simulink model "Hector_Simulation"  (R2023b)
settings: Solver=daessc  StartTime=0.0  StopTime=Tf  FixedStep=0.001  MaxStep=1e-3  RelTol=1e-2
model workspace (MATLAB code in the model file):
  | %% World Plane
  | plane_x = 20;
  | plane_y = 2;
  | plane_z = 0.05;
  | 
  | %% motor
  | %A1
  | motor_com = [0, -0.02,0];
  | motor_com_mirror = [0, 0.02,0];
  | 
  | motor_I = [0.00048,0.00071,0.00048];
  | motor_mass = 0.605;
  | 
  | %% Body
  | % Inertial
  | body_com_x = 0.0;
  | body_com_y = 0.0;
  | body_com_z = -0.0;
  | body_mass = 5.75;
  | body_ixx = 44350*1e-6;
  | body_ixy = 0.0;
  | body_ixz = 0.0;
  | body_iyy = 53149*1e-6;
  | body_iyz = 0.0;
  | body_izz = 21390*1e-6;
  | 
  | %% Hip 1
  | % joint
  | hip1_offset_x =0.0;
  | hip1_offset_y = 0.047;
  | hip1_offset_z = 0.1265;
  | % hip1_max = 15;
  | % hip1_min = -15;
  | hip1_velocity_max = 21;
  | hip1_torque_max = 33.5;
  | % Inertial
  | hip1_com_x = 0.0268;
  | hip1_com_y = -0.00315;
  | hip1_com_z = -0.0272;
  | hip1_mass = 0.173;
  | hip1_ixx = 0.00022;
  | hip1_ixy = 0.0;
  | hip1_ixz = 0.0;
  | hip1_iyy = 0.00024;
  | hip1_iyz = 0.0;
  | hip1_izz = 0.00016;
  | 
  | %% Hip 2
  | % joint
  | hip2_offset_x =0.053;
  | hip2_offset_y = 0.0185;
  | hip2_offset_z = 0.071;
  | % hip2_max = 15;
  | % hip2_min = -15;
  | hip2_velocity_max = 21;
  | hip2_torque_max = 33.5;
  | % Inertial
  | hip2_com_x = -0.0308;
  | hip2_com_y = -0.00942;
  | hip2_com_z = 0.0;
  | hip2_mass = 0.0722;
  | hip2_ixx = 0.0000422;
  | hip2_ixy = 0.0;
  | hip2_ixz = 0.0;
  | hip2_iyy = 0.000120;
  | hip2_iyz = 0.0;
  | hip2_izz = 0.0000708;
  | 
  | %% Thigh
  | % joint
  | thigh_offset_x =-0.06;
  | thigh_offset_y = 0.004;
  | thigh_offset_z = 0.0;
  | % thigh_max = 130;
  | % thigh_min = -45;
  | thigh_velocity_max = 21;
  | thigh_torque_max = 33.5;
  | % Inertial
  | thigh_com_x = -0.00143;
  | thigh_com_y = -0.02106;
  | thigh_com_z = -0.06115;
  | thigh_mass = 0.397;
  | thigh_ixx = 0.00197;
  | thigh_ixy = 0.0;
  | thigh_ixz = 0.0;
  | thigh_iyy = 0.00218;
  | thigh_iyz = 0.0;
  | thigh_izz = 0.00033;
  | 
  | ankle_motor_offset_x = 0;
  | ankle_motor_offset_y = 0.039;
  | ankle_motor_offset_z = 0;
  | 
  | knee_motor_offset_x = 0;
  | knee_motor_offset_y = 0.039;
  | knee_motor_offset_z = -0.095;
  | 
  | %% Calf
  | % joint
  | calf_offset_x = 0.0;
  | calf_offset_y = 0.003;
  | calf_offset_z = -0.22;
  | % calf_max = 0;
  | % calf_min = -135;
  | % knee_max = 0;
  | % knee_min = -160;
  | calf_velocity_max = 14*1.5;
  | calf_torque_max = 51;
  | % Inertial
  | calf_com_x = 0.00165;
  | calf_com_y = -0.01117;
  | calf_com_z = -0.06438;
  | calf_mass = 0.136;
  | calf_ixx = 0.00071;
  | calf_ixy = 0.0;
  | calf_ixz = 0.0;
  | calf_iyy = 0.00072;
  | calf_iyz = 0.0;
  | calf_izz = 0.00002;
  | 
  | %% Toe
  | % joint
  | toe_offset_x = 0.0;
  | toe_offset_y = 0.011;
  | toe_offset_z = -0.22;
  | % toe_max = 60;
  | % toe_min = -60;
  | toe_velocity_max = 21;
  | toe_torque_max = 33.5;
  | % Inertial
  | toe_com_x = 0.00239;
  | toe_com_y = 0.00002;
  | toe_com_z = -0.02261;
  | toe_mass = 0.08425;
  | toe_ixx = 0.00001;
  | toe_ixy = 0.0;
  | toe_ixz = 0.0;
  | toe_iyy = 0.00011;
  | toe_iyz = 0.0;
  | toe_izz = 0.00011;
  | %% Contact
  | contact_front = 0.091;
  | contact_rear = -0.061;
  | contact_right = 0.026;
  | contact_left = 0.01;
  | contact_z = 0.039;
  | 
  | %%
  | %dorito
  | dorito_offset_x = 0;
  | dorito_offset_y = 0.012;
  | dorito_offset_z = 0;
  | 
  | dorito_lower_connection = [0.034 0 -0.044];
  | dorito_upper_connection = [0.034 0 0.021];
  | 
  | linkage_mass = 0.051;
  | linkage_com = [0 0 -0.11];
  | linkage_I = [0.00001 0.00002 0.00002];
  | %% Arms
  | shoulder_com_x = 0;
  | shoulder_com_y = 0;
  | shoulder_com_z = 0;
  | shoulder_mass = 0.835;
  | % shoulder_mass = 0.05;
  | shoulder_ixx = 920*1e-6;
  | shoulder_ixy = 0.0;
  | shoulder_ixz = 0.0;
  | shoulder_iyy = 270*1e-6;
  | shoulder_iyz = 0.0;
  | shoulder_izz = 499*1e-6;
  | 
  | upperarm_com_x = 0;
  | upperarm_com_y = 0;
  | upperarm_com_z = 0;
  | upperarm_mass = 1.35;
  | % upperarm_mass = 0.05;
  | upperarm_ixx = 1200*1e-6;
  | upperarm_ixy = 0.0;
  | upperarm_ixz = 0.0;
  | upperarm_iyy = 1170*1e-6;
  | upperarm_iyz = 0.0;
  | upperarm_izz = 729*1e-6;
  | 
  | forearm_com_x = 0;
  | forearm_com_y = 0;
  | forearm_com_z = -0.10;
  | forearm_mass = 0.53;
  | % forearm_mass = 0.03;
  | forearm_ixx = 427*1e-6;
  | forearm_ixy = 0.0;
  | forearm_ixz = 0.0;
  | forearm_iyy = 466*1e-6;
  | forearm_iyz = 0.0;
  | forearm_izz = 72*1e-6;
values from neighbouring files (symbols this model uses):
  Tf = 5    [createNeuralNetworksOptions.m]
  Ts = 0.04    [createNeuralNetworksOptions.m]
undefined symbols (not defined in the file or in its folder): body_v0, body_z0, init_height, sigbuilder_block, X, Y, Z
libraries: sm_lib x134, nesl_utility x77, simulink x8, walkingRobotUtils x1, rllib x1
(part 2 of 6)

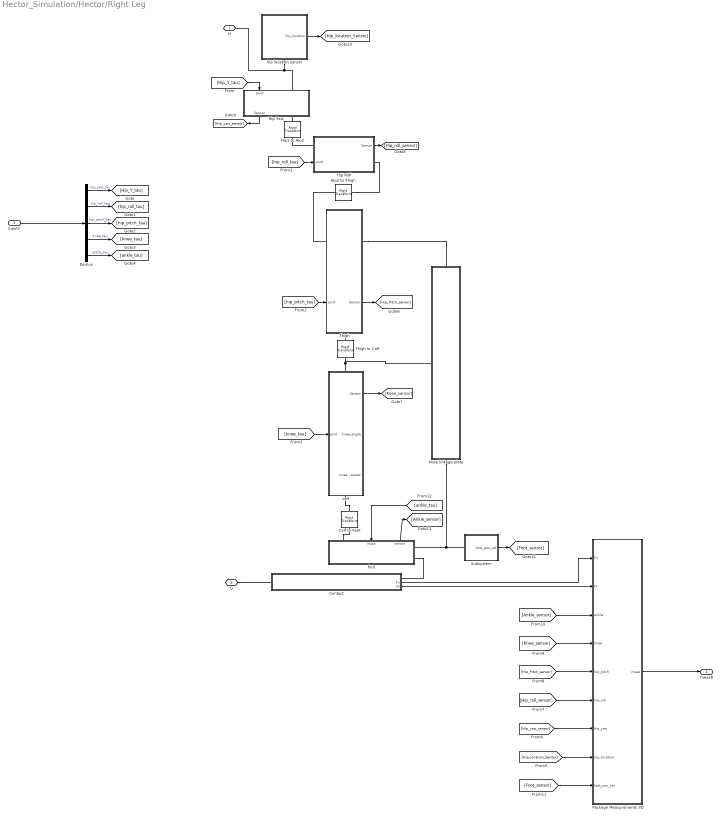
== system Hector_Simulation/Hector/Right Leg ==
  Inputs : Inport
  Calf to Feet : sm_lib/Frames and Transforms/Rigid Transform  TranslationMethod=Cartesian  TranslationStandardOffset=0  TranslationStandardOffsetUnits=m  TranslationStandardAxis=+Z  TranslationCartesianOffset=[toe_offset_x -toe_offset_y toe_offset_z]  TranslationCartesianOffsetUnits=m  TranslationROffset=0  TranslationROffsetUnits=m  TranslationZOffset=0  TranslationZOffsetUnits=m  TranslationThetaOffset=0  TranslationThetaOffsetUnits=deg  RotationMethod=StandardAxis  RotationAngleUnits=deg  RotationStandardAxis=-X  RotationAngle=90  RotationArbitraryAxis=[0 0 1]  FollAlignAxisA=+X  BaseAlignAxisA=+Y  FollAlignAxisB=+Y  BaseAlignAxisB=+Z  RotationSequenceAxes=FollowerAxes  RotationSequence=XYX  RotationSequenceAngles=[0 0 0]  RotationSequenceAnglesUnits=deg  RotationMatrix=[1 0 0; 0 1 0; 0 0 1]  Quaternion=[1 0 0 0]
  Contact : Subsystem
      settings: PortSchema="{\"entries\":[{\"content\":{\"sides\":[{\"content\":{},\"type\":\"ConnectorPlacement.EquallySpacedRectSide\",\"uuid\":\"90cb039b-e836-4135-af72-350f65081789\"},{\"content\":{\"side\":\"RIGHT\"},\"type\":\"ConnectorPlacement.EquallySpacedRectSide\",\"uuid\":\"81d48f4c-41f3-4d90-8a93-e0d0a46d5b2e\"},{\"content\":{\"connectorIds\":[\"LConn1\"],\"side\":\"TOP\"},\"type\":\"ConnectorPlacement.EquallySpacedRectSide\",\"uuid\":\"b67ccfe2-cb2a-4099-b095-526df9395d8f\"},{\"content\":{\"connectorIds\":[\"Out1\",\"Out2\",\"RConn1\"],\"side\":\"BOTTOM\"},\"type\":\"ConnectorPlacement.EquallySpacedRectSide\",\"uuid\":\"6caa8e19-1421-4e04-b7b7-5a566660e146\"}]},\"type\":\"ConnectorPlacement.EquallySpacedConnector\",\"uuid\":\"53598f80-6515-4118-9b20-e27054ed147b\"}],\"packageUris\":[\"http://schema.mathworks.com/mf0/Connector/R2020b\"],\"version\":\"1.0\"}"
  Demux : Demux  Outputs=5
  "Hip Roll " : Subsystem
      settings: PortSchema="{\"entries\":[{\"content\":{\"sides\":[{\"content\":{\"connectorIds\":[\"LConn1\",\"In1\"]},\"type\":\"ConnectorPlacement.EquallySpacedRectSide\",\"uuid\":\"f10cd686-4b19-42e5-8833-cb4a27185591\"},{\"content\":{\"connectorIds\":[\"Out1\",\"RConn1\"],\"side\":\"RIGHT\"},\"type\":\"ConnectorPlacement.EquallySpacedRectSide\",\"uuid\":\"54dd9d3c-113c-45fd-a52f-bea50d6d1d07\"},{\"content\":{\"side\":\"TOP\"},\"type\":\"ConnectorPlacement.EquallySpacedRectSide\",\"uuid\":\"b1bd9e47-98e3-4c50-90f2-eee15cbac121\"}]},\"type\":\"ConnectorPlacement.EquallySpacedConnector\",\"uuid\":\"7e05ec0b-e972-4059-8004-c87e94cf3608\"}],\"packageUris\":[\"http://schema.mathworks.com/mf0/Connector/R2020b\"],\"version\":\"1.0\"}"
  "Hip Yaw " : Subsystem
      settings: PortSchema="{\"entries\":[{\"content\":{\"sides\":[{\"content\":{\"connectorIds\":[\"LConn1\",\"In1\"]},\"type\":\"ConnectorPlacement.EquallySpacedRectSide\",\"uuid\":\"f10cd686-4b19-42e5-8833-cb4a27185591\"},{\"content\":{\"connectorIds\":[\"RConn1\",\"Out1\"],\"side\":\"RIGHT\"},\"type\":\"ConnectorPlacement.EquallySpacedRectSide\",\"uuid\":\"54dd9d3c-113c-45fd-a52f-bea50d6d1d07\"},{\"content\":{\"side\":\"TOP\"},\"type\":\"ConnectorPlacement.EquallySpacedRectSide\",\"uuid\":\"b1bd9e47-98e3-4c50-90f2-eee15cbac121\"}]},\"type\":\"ConnectorPlacement.EquallySpacedConnector\",\"uuid\":\"7e05ec0b-e972-4059-8004-c87e94cf3608\"}],\"packageUris\":[\"http://schema.mathworks.com/mf0/Connector/R2020b\"],\"version\":\"1.0\"}"
  Hip1 to Hip2 : sm_lib/Frames and Transforms/Rigid Transform  TranslationMethod=Cartesian  TranslationStandardOffset=0  TranslationStandardOffsetUnits=m  TranslationStandardAxis=+Z  TranslationCartesianOffset=[hip2_offset_x-0.014 -hip2_offset_y -hip2_offset_z]  TranslationCartesianOffsetUnits=m  TranslationROffset=0  TranslationROffsetUnits=m  TranslationZOffset=0  TranslationZOffsetUnits=m  TranslationThetaOffset=0  TranslationThetaOffsetUnits=deg  RotationMethod=StandardAxis  RotationAngleUnits=deg  RotationStandardAxis=+Y  RotationAngle=90  RotationArbitraryAxis=[0 0 1]  FollAlignAxisA=+X  BaseAlignAxisA=+Y  FollAlignAxisB=+Y  BaseAlignAxisB=+Z  RotationSequenceAxes=FollowerAxes  RotationSequence=XYX  RotationSequenceAngles=[0 0 0]  RotationSequenceAnglesUnits=deg  RotationMatrix=[1 0 0; 0 1 0; 0 0 1]  Quaternion=[1 0 0 0]
  Hip2 to Thigh : sm_lib/Frames and Transforms/Rigid Transform  TranslationMethod=Cartesian  TranslationStandardOffset=0  TranslationStandardOffsetUnits=m  TranslationStandardAxis=+Z  TranslationCartesianOffset=[thigh_offset_x -thigh_offset_y-0.014 thigh_offset_z]  TranslationCartesianOffsetUnits=m  TranslationROffset=0  TranslationROffsetUnits=m  TranslationZOffset=0  TranslationZOffsetUnits=m  TranslationThetaOffset=0  TranslationThetaOffsetUnits=deg  RotationMethod=StandardAxis  RotationAngleUnits=deg  RotationStandardAxis=-X  RotationAngle=90  RotationArbitraryAxis=[0 0 1]  FollAlignAxisA=+X  BaseAlignAxisA=+Y  FollAlignAxisB=+Y  BaseAlignAxisB=+Z  RotationSequenceAxes=FollowerAxes  RotationSequence=XYX  RotationSequenceAngles=[0 0 0]  RotationSequenceAnglesUnits=deg  RotationMatrix=[1 0 0; 0 1 0; 0 0 1]  Quaternion=[1 0 0 0]
  Knee linkage plate : Subsystem
      settings: PortSchema="{\"entries\":[{\"content\":{\"sides\":[{\"content\":{\"connectorIds\":[\"LConn1\"]},\"type\":\"ConnectorPlacement.EquallySpacedRectSide\",\"uuid\":\"d15cbd26-48d6-4124-8c9e-86308e1b9742\"},{\"content\":{\"side\":\"RIGHT\"},\"type\":\"ConnectorPlacement.EquallySpacedRectSide\",\"uuid\":\"1775c2f6-8f0d-46c0-b772-c53e3201c4d6\"},{\"content\":{\"connectorIds\":[\"LConn2\"],\"side\":\"TOP\"},\"type\":\"ConnectorPlacement.EquallySpacedRectSide\",\"uuid\":\"48d307f9-6320-48e8-908a-f6f6021bd930\"},{\"content\":{\"connectorIds\":[\"RConn1\"],\"side\":\"BOTTOM\"},\"type\":\"ConnectorPlacement.EquallySpacedRectSide\",\"uuid\":\"b3c67006-0b54-4332-92d7-051cc1bfd2ae\"}]},\"type\":\"ConnectorPlacement.EquallySpacedConnector\",\"uuid\":\"60bd5e18-277f-4e49-aed3-720673bccfc7\"}],\"packageUris\":[\"http://schema.mathworks.com/mf0/Connector/R2020b\"],\"version\":\"1.0\"}"
  Package Measurements 3D : Subsystem  AncestorBlock=walkingRobotUtils/Package Measurements 3D
      settings: LibrarySourceBlock=|
      | walkingRobotUtils/Package
      | Measurements 3D
  Subsystem : Subsystem
  Thigh : Subsystem
      settings: PortSchema="{\"entries\":[{\"content\":{\"sides\":[{\"content\":{\"connectorIds\":[\"LConn1\",\"In1\"]},\"type\":\"ConnectorPlacement.EquallySpacedRectSide\",\"uuid\":\"f10cd686-4b19-42e5-8833-cb4a27185591\"},{\"content\":{\"connectorIds\":[\"RConn1\",\"Out1\"],\"side\":\"RIGHT\"},\"type\":\"ConnectorPlacement.EquallySpacedRectSide\",\"uuid\":\"54dd9d3c-113c-45fd-a52f-bea50d6d1d07\"},{\"content\":{\"side\":\"TOP\"},\"type\":\"ConnectorPlacement.EquallySpacedRectSide\",\"uuid\":\"b1bd9e47-98e3-4c50-90f2-eee15cbac121\"},{\"content\":{\"connectorIds\":[\"RConn2\"],\"side\":\"BOTTOM\"},\"type\":\"ConnectorPlacement.EquallySpacedRectSide\",\"uuid\":\"56668063-a02b-4ab1-95ca-0037226f6e4e\"}]},\"type\":\"ConnectorPlacement.EquallySpacedConnector\",\"uuid\":\"7e05ec0b-e972-4059-8004-c87e94cf3608\"}],\"packageUris\":[\"http://schema.mathworks.com/mf0/Connector/R2020b\"],\"version\":\"1.0\"}"
  Thigh to Calf : sm_lib/Frames and Transforms/Rigid Transform  TranslationMethod=Cartesian  TranslationStandardOffset=0  TranslationStandardOffsetUnits=m  TranslationStandardAxis=+Z  TranslationCartesianOffset=[calf_offset_x -calf_offset_y calf_offset_z]  TranslationCartesianOffsetUnits=m  TranslationROffset=0  TranslationROffsetUnits=m  TranslationZOffset=0  TranslationZOffsetUnits=m  TranslationThetaOffset=0  TranslationThetaOffsetUnits=deg  RotationMethod=StandardAxis  RotationAngleUnits=deg  RotationStandardAxis=-X  RotationAngle=90  RotationArbitraryAxis=[0 0 1]  FollAlignAxisA=+X  BaseAlignAxisA=+Y  FollAlignAxisB=+Y  BaseAlignAxisB=+Z  RotationSequenceAxes=FollowerAxes  RotationSequence=XYX  RotationSequenceAngles=[0 0 0]  RotationSequenceAnglesUnits=deg  RotationMatrix=[1 0 0; 0 1 0; 0 0 1]  Quaternion=[1 0 0 0]
  calf : Subsystem
      settings: PortSchema="{\"entries\":[{\"content\":{\"sides\":[{\"content\":{\"connectorIds\":[\"In1\"]},\"type\":\"ConnectorPlacement.EquallySpacedRectSide\",\"uuid\":\"eea5befc-3e1f-4115-922f-c8b9a985aa8c\"},{\"content\":{\"connectorIds\":[\"Out1\",\"Out2\",\"Out3\"],\"side\":\"RIGHT\"},\"type\":\"ConnectorPlacement.EquallySpacedRectSide\",\"uuid\":\"cbd2e1ae-207a-4bb1-94cd-07f8d3cfb935\"},{\"content\":{\"connectorIds\":[\"LConn1\"],\"side\":\"TOP\"},\"type\":\"ConnectorPlacement.EquallySpacedRectSide\",\"uuid\":\"a7ce038b-3340-4913-81e9-0867ebf4655c\"},{\"content\":{\"connectorIds\":[\"RConn1\"],\"side\":\"BOTTOM\"},\"type\":\"ConnectorPlacement.EquallySpacedRectSide\",\"uuid\":\"74c932de-4238-43ff-bcae-b7ffce22b182\"}]},\"type\":\"ConnectorPlacement.EquallySpacedConnector\",\"uuid\":\"77d8afa2-2f83-4e63-811f-f6c2ad6c93b0\"}],\"packageUris\":[\"http://schema.mathworks.com/mf0/Connector/R2020b\"],\"version\":\"1.0\"}"
  foot : Subsystem
      settings: PortSchema="{\"entries\":[{\"content\":{\"sides\":[{\"content\":{},\"type\":\"ConnectorPlacement.EquallySpacedRectSide\",\"uuid\":\"db4923ac-49b4-42e1-b40d-7661ce4f57bd\"},{\"content\":{\"connectorIds\":[\"RConn1\",\"RConn2\"],\"side\":\"RIGHT\"},\"type\":\"ConnectorPlacement.EquallySpacedRectSide\",\"uuid\":\"09705837-effb-467f-b653-050bef978399\"},{\"content\":{\"connectorIds\":[\"LConn1\",\"In1\",\"Out1\"],\"side\":\"TOP\"},\"type\":\"ConnectorPlacement.EquallySpacedRectSide\",\"uuid\":\"4080e974-ebe1-4132-a69c-8d3e8f98addf\"}]},\"type\":\"ConnectorPlacement.EquallySpacedConnector\",\"uuid\":\"6a0abf02-e0ef-449a-af3b-6b2ef388d347\"}],\"packageUris\":[\"http://schema.mathworks.com/mf0/Connector/R2020b\"],\"version\":\"1.0\"}"
  hip location sensor : Subsystem
      settings: PortSchema="{\"entries\":[{\"content\":{\"sides\":[{\"content\":{},\"type\":\"ConnectorPlacement.EquallySpacedRectSide\",\"uuid\":\"56b65547-b272-4cdf-b2ea-30862c141d1b\"},{\"content\":{\"connectorIds\":[\"Out1\"],\"side\":\"RIGHT\"},\"type\":\"ConnectorPlacement.EquallySpacedRectSide\",\"uuid\":\"1d3a1f86-712b-4a8c-acf9-2be1a05e74d9\"},{\"content\":{\"side\":\"TOP\"},\"type\":\"ConnectorPlacement.EquallySpacedRectSide\",\"uuid\":\"85a20169-add0-4c5e-91a2-5f372731ee54\"},{\"content\":{\"connectorIds\":[\"RConn1\"],\"side\":\"BOTTOM\"},\"type\":\"ConnectorPlacement.EquallySpacedRectSide\",\"uuid\":\"ec32ff90-c4af-429b-bf57-0a5f431ccab7\"}]},\"type\":\"ConnectorPlacement.EquallySpacedConnector\",\"uuid\":\"6514ea8e-2609-4bc5-b886-24d268738c3d\"}],\"packageUris\":[\"http://schema.mathworks.com/mf0/Connector/R2020b\"],\"version\":\"1.0\"}"
  H : PMIOPort  Side=Left
  G : PMIOPort  Port=2  Side=Right
  measR : Outport  VectorParamsAs1DForOutWhenUnconnected=off
  wires:
  [Foot_sensor] -> Package Measurements 3D/9(foot_pos_vel)
  "Hip Roll "/1(Sensor) -> [Hip_roll_sensor]
  Demux/4 -> [knee_tau]  "knee_tau"
  [Knee_sensor] -> Package Measurements 3D/4(knee)
  calf/1(Sensor) -> [Knee_sensor]
  [Hip_Pitch_sensor] -> Package Measurements 3D/5(hip_pitch)
  Demux/5 -> [ankle_tau]  "ankle_tau"
  [Ankle_sensor] -> Package Measurements 3D/3(ankle)
  [Hip_roll_sensor] -> Package Measurements 3D/6(hip_roll)
  [Hip_yaw_sensor] -> Package Measurements 3D/7(hip_yaw)
  foot/1(sensor) -> [Ankle_sensor]
  Subsystem/1(foot_pos_vel) -> [Foot_sensor]
  [hip_roll_tau] -> "Hip Roll "/1(joint)
  "Hip Yaw "/1(Sensor) -> [Hip_yaw_sensor]
  Demux/1 -> [Hip_Y_tau]  "hip_yaw_tau"
  [knee_tau] -> calf/1(Joint)
  hip location sensor/1(hip_location) -> [Hip_location_Sensor]
  Demux/3 -> [hip_pitch_tau]  "hip_pitch_tau"
  [Hip_location_Sensor] -> Package Measurements 3D/8(hip_location)
  [ankle_tau] -> foot/1(input)
  [Hip_Y_tau] -> "Hip Yaw "/1(Joint)
  [hip_pitch_tau] -> Thigh/1(Joint)
  Inputs/1 -> Demux/1
  Contact/2(Fn) -> Package Measurements 3D/1(Fn)
  Thigh/1(Sensor) -> [Hip_Pitch_sensor]
  Contact/1(Ff) -> Package Measurements 3D/2(Ff)
  Demux/2 -> [hip_roll_tau]  "hip_roll_tau"
  Package Measurements 3D/1(meas) -> measR/1
  connections:
  H/RConn1 -- hip location sensor/RConn1 -- "Hip Yaw "/LConn1
  Thigh to Calf/RConn1 -- Knee linkage plate/LConn1 -- calf/LConn1
  foot/RConn1 -- Subsystem/LConn1 -- Knee linkage plate/RConn1
  foot/LConn1 -- Calf to Feet/RConn1
  Thigh/RConn1 -- Knee linkage plate/LConn2
  calf/RConn1 -- Calf to Feet/LConn1
  Thigh/LConn1 -- Hip2 to Thigh/RConn1
  G/RConn1 -- Contact/LConn1
  Thigh to Calf/LConn1 -- Thigh/RConn2
  Hip1 to Hip2/LConn1 -- "Hip Yaw "/RConn1
  "Hip Roll "/LConn1 -- Hip1 to Hip2/RConn1
  Hip2 to Thigh/LConn1 -- "Hip Roll "/RConn1
  foot/RConn2 -- Contact/RConn1

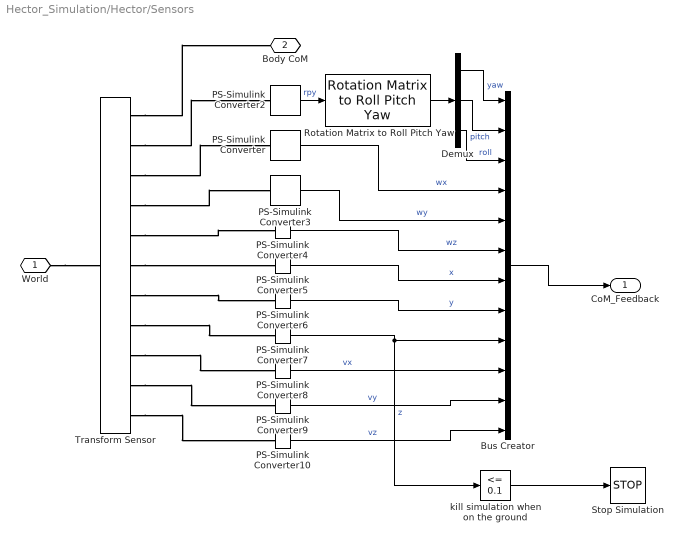
== system Hector_Simulation/Hector/Sensors ==
  Bus Creator : BusCreator  Inputs=12
  Demux : Demux  Outputs=3
  PS-Simulink Converter : nesl_utility/PS-Simulink Converter  PhysicalDomain=network_engine_domain  SubClassName=ps_output  LeftPortType=input  RightPortType=output  PseudoPeriodic=off  Frequencies=[]  VectorFormat=1-D array  Unit=1  AffineConversion=off
  PS-Simulink Converter{3..10} (8 alike) : nesl_utility/PS-Simulink Converter  PhysicalDomain=network_engine_domain  SubClassName=ps_output  LeftPortType=input  RightPortType=output  PseudoPeriodic=off  Frequencies=[]  VectorFormat=1-D array  Unit=inherit  AffineConversion=off
  PS-Simulink Converter2 : nesl_utility/PS-Simulink Converter  PhysicalDomain=network_engine_domain  SubClassName=ps_output  LeftPortType=input  RightPortType=output  PseudoPeriodic=off  Frequencies=[]  VectorFormat=1-D array  Unit=1  AffineConversion=off
  Rotation Matrix to Roll Pitch Yaw : walkingRobotUtils/Rotation Matrix to  Roll Pitch Yaw  SystemSampleTime=-1  VariantActivationTime=update diagram  AllowFlexibleInterface=on  Latency=0  AutoFrameSizeCalculation=off
  Stop Simulation : Stop
  Transform Sensor : sm_lib/Frames and Transforms/Transform Sensor  MeasurementFrame=World  RotationSequence=XYZ  SenseAngle=off  SenseAxis=off  SenseQ=off  SenseR=off  SenseRotationSequence=on  SenseOmegaX=on  SenseOmegaY=on  SenseOmegaZ=on  SenseOmega=off  SenseQDot=off  SenseRDot=off  SenseRotationSequenceDot=off  SenseAlphaX=off  SenseAlphaY=off  SenseAlphaZ=off  SenseAlpha=off  SenseQDDot=off  SenseRDDot=off  SenseX=on  SenseY=on  SenseZ=on  SenseXYZ=off  SenseRad=off  SenseAzim=off  SenseDist=off  SenseInc=off  SenseXDot=on  SenseYDot=on  SenseZDot=on  SenseXYZDot=off  SenseRadDot=off  SenseAzimDot=off  SenseDistDot=off  SenseIncDot=off  SenseXDDot=off  SenseYDDot=off  SenseZDDot=off  SenseXYZDDot=off  SenseRadDDot=off  SenseAzimDDot=off  SenseDistDDot=off  SenseIncDDot=off
  kill simulation when on the ground : simulink/Logic and Bit Operations/Compare To Constant  relop=<=  const=0.1  OutDataTypeStr=boolean
  World : PMIOPort  Side=Left
  Body CoM : PMIOPort  Port=2  Side=Right
  CoM_Feedback : Outport
  wires:
  PS-Simulink Converter7/1 -> Bus Creator/9, kill simulation when on the ground/1  "z"
  Bus Creator/1 -> CoM_Feedback/1
  kill simulation when on the ground/1 -> Stop Simulation/1
  PS-Simulink Converter2/1 -> Rotation Matrix to Roll Pitch Yaw/1  "rpy"
  Rotation Matrix to Roll Pitch Yaw/1 -> Demux/1
  Demux/1 -> Bus Creator/1  "yaw"
  Demux/2 -> Bus Creator/2  "pitch"
  Demux/3 -> Bus Creator/3  "roll"
  PS-Simulink Converter/1 -> Bus Creator/4  "wx"
  PS-Simulink Converter3/1 -> Bus Creator/5  "wy"
  PS-Simulink Converter4/1 -> Bus Creator/6  "wz"
  PS-Simulink Converter5/1 -> Bus Creator/7  "x"
  PS-Simulink Converter6/1 -> Bus Creator/8  "y"
  PS-Simulink Converter8/1 -> Bus Creator/10  "vx"
  PS-Simulink Converter9/1 -> Bus Creator/11  "vy"
  PS-Simulink Converter10/1 -> Bus Creator/12  "vz"
  connections:
  World/RConn1 -- Transform Sensor/LConn1
  Transform Sensor/RConn7 -- PS-Simulink Converter6/LConn1
  Transform Sensor/RConn5 -- PS-Simulink Converter4/LConn1
  Transform Sensor/RConn3 -- PS-Simulink Converter/LConn1
  Transform Sensor/RConn1 -- Body CoM/RConn1
  Transform Sensor/RConn6 -- PS-Simulink Converter5/LConn1
  Transform Sensor/RConn4 -- PS-Simulink Converter3/LConn1
  Transform Sensor/RConn2 -- PS-Simulink Converter2/LConn1
  Transform Sensor/RConn8 -- PS-Simulink Converter7/LConn1
  Transform Sensor/RConn9 -- PS-Simulink Converter8/LConn1
  Transform Sensor/RConn10 -- PS-Simulink Converter9/LConn1
  Transform Sensor/RConn11 -- PS-Simulink Converter10/LConn1

== system Hector_Simulation/Hector/external force x ==
  Demux : Demux  Tag=STV Demux  Outputs=1
      settings: DisplayOption=none
  FromWs : FromWorkspace  Tag=STV FromWs  VariableName=tuvar
      SigBuilderData=|
      | common.afterFinalStr = 'Extrapolate'
      | common.sampleTime = 0
      | dataSet.timeRange = [0 10]
      | dataSet.name = 'Group 1'
      | sbobj.Groups.Name = 'Group 1'
      | sbobj.Groups.Signals.Name = 'Signal 1'
      | sbobj.Groups.Signals.XData = [0 0.5 0.6 0.7 10]
      | sbobj.Groups.Signals.YData = [0 0 90 0 0]
  Signal 1 : Outport  Tag=STV Outport
  wires:
  Demux/1 -> Signal 1/1
  FromWs/1 -> Demux/1

== system Hector_Simulation/Hector/external force y ==
  Demux : Demux  Tag=STV Demux  Outputs=1
      settings: DisplayOption=none
  FromWs : FromWorkspace  Tag=STV FromWs  VariableName=tuvar
      SigBuilderData=|
      | common.afterFinalStr = 'Extrapolate'
      | common.sampleTime = 0
      | dataSet.timeRange = [0 10]
      | dataSet.name = 'Group 1'
      | sbobj.Groups.Name = 'Group 1'
      | sbobj.Groups.Signals.Name = 'Signal 1'
      | sbobj.Groups.Signals.XData = [0 1 1.1 1.2 10]
      | sbobj.Groups.Signals.YData = [0 0 70 0 0]
  Signal 1 : Outport  Tag=STV Outport
  wires:
  Demux/1 -> Signal 1/1
  FromWs/1 -> Demux/1

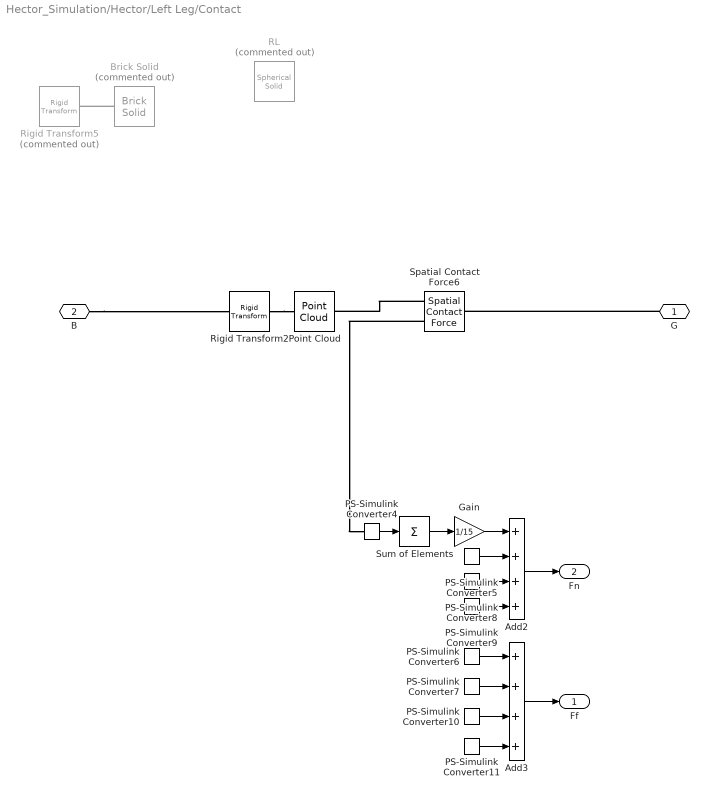
== system Hector_Simulation/Hector/Left Leg/Contact ==
  Add2 : Sum  Inputs=++++
  Add3 : Sum  Inputs=++++
  Brick Solid : sm_lib/Body Elements/Brick Solid  Commented=on  GraphicAmbientColor=[0.15 0.15 0.15 1.0]  BasedOnType=Density  BrickDimensions=[0.16 0.02 0.0001]  BrickDimensionsUnits=m  CenterOfMass=[0 0 0]  CenterOfMassUnits=m  GraphicDiffuseColor=[0.5 0.5 0.5]  Density=1000  DensityUnits=kg/m^3  DoExposeReferenceFrame=on  GraphicEmissiveColor=[0.0 0.0 0.0 1.0]  ExportEntireGeometry=on  SerializedFrames=<Frames/>  MarkerShape=Sphere  MarkerSize=10  GraphicType=FromGeometry  InertiaType=PointMass  Mass=0  MassUnits=kg  MomentsOfInertia=[1 1 1]  MomentsOfInertiaUnits=kg*m^2  GraphicOpacity=1.0  ProductsOfInertia=[0 0 0]  ProductsOfInertiaUnits=kg*m^2  GraphicShininess=75  GraphicSpecularColor=[0.5 0.5 0.5 1.0]  GraphicVisPropType=SimpleVisualProperties
  Gain : Gain  Gain=1/15
  PS-Simulink Converter{4..11} (8 alike) : nesl_utility/PS-Simulink Converter  PhysicalDomain=network_engine_domain  SubClassName=ps_output  LeftPortType=input  RightPortType=output  PseudoPeriodic=off  Frequencies=[]  VectorFormat=1-D array  Unit=inherit  AffineConversion=off
  Point Cloud : sm_lib/Curves and Surfaces/Point Cloud  CoordinatesMatrix=contact_cloud  CoordinatesMatrixUnits=m  GraphicType=MarkerCloud  GraphicSphereRadius=0.001  GraphicSphereRadiusUnits=m  GraphicVisPropType=SimpleVisualProperties  GraphicDiffuseColor=[0.5 0.5 0.5]  GraphicOpacity=1.0  GraphicSpecularColor=[0.5 0.5 0.5 1.0]  GraphicAmbientColor=[0.15 0.15 0.15 1.0]  GraphicEmissiveColor=[0.0 0.0 0.0 1.0]  GraphicShininess=75
  RL : sm_lib/Body Elements/Spherical Solid  Commented=on  GraphicAmbientColor=[0.15 0.15 0.15 1.0]  BasedOnType=Density  CenterOfMass=[0 0 0]  CenterOfMassUnits=m  GraphicDiffuseColor=[1.0 0.0 0.2]  Density=0  DensityUnits=kg/m^3  DoExposeReferenceFrame=on  GraphicEmissiveColor=[0.0 0.0 0.0 1.0]  ExportEntireGeometry=on  SerializedExposedGeometries=<ExposedGeometries><ExposedGeometry><RawGeometryId>entire</RawGeometryId><ExposedGeometryId>G</ExposedGeometryId></ExposedGeometry></ExposedGeometries>  SerializedFrames=<Frames/>  MarkerShape=Sphere  MarkerSize=10  GraphicType=FromGeometry  InertiaType=CalculateFromGeometry  Mass=1  MassUnits=kg  MomentsOfInertia=[1 1 1]  MomentsOfInertiaUnits=kg*m^2  GraphicOpacity=1.0  ProductsOfInertia=[0 0 0]  ProductsOfInertiaUnits=kg*m^2  GraphicShininess=75  GraphicSpecularColor=[0.5 0.5 0.5 1.0]  SphereRadius=contact_point_radius  SphereRadiusUnits=m  GraphicVisPropType=SimpleVisualProperties
  Rigid Transform2 : sm_lib/Frames and Transforms/Rigid Transform  TranslationMethod=Cartesian  TranslationStandardOffset=0  TranslationStandardOffsetUnits=m  TranslationStandardAxis=+Z  TranslationCartesianOffset=[0 0.0 -contact_z]  TranslationCartesianOffsetUnits=m  TranslationROffset=0  TranslationROffsetUnits=m  TranslationZOffset=0  TranslationZOffsetUnits=m  TranslationThetaOffset=0  TranslationThetaOffsetUnits=deg  RotationMethod=None  RotationAngleUnits=deg  RotationStandardAxis=+Z  RotationAngle=0.0  RotationArbitraryAxis=[0 0 1]  FollAlignAxisA=+X  BaseAlignAxisA=+Y  FollAlignAxisB=+Y  BaseAlignAxisB=+Z  RotationSequenceAxes=FollowerAxes  RotationSequence=XYX  RotationSequenceAngles=[0 0 0]  RotationSequenceAnglesUnits=deg  RotationMatrix=[1 0 0; 0 1 0; 0 0 1]  Quaternion=[1 0 0 0]
  Rigid Transform5 : sm_lib/Frames and Transforms/Rigid Transform  Commented=on  TranslationMethod=Cartesian  TranslationStandardOffset=0  TranslationStandardOffsetUnits=m  TranslationStandardAxis=+Z  TranslationCartesianOffset=[0.015 2*contact_left -contact_z]  TranslationCartesianOffsetUnits=m  TranslationROffset=0  TranslationROffsetUnits=m  TranslationZOffset=0  TranslationZOffsetUnits=m  TranslationThetaOffset=0  TranslationThetaOffsetUnits=deg  RotationMethod=None  RotationAngleUnits=deg  RotationStandardAxis=+Z  RotationAngle=0.0  RotationArbitraryAxis=[0 0 1]  FollAlignAxisA=+X  BaseAlignAxisA=+Y  FollAlignAxisB=+Y  BaseAlignAxisB=+Z  RotationSequenceAxes=FollowerAxes  RotationSequence=XYX  RotationSequenceAngles=[0 0 0]  RotationSequenceAnglesUnits=deg  RotationMatrix=[1 0 0; 0 1 0; 0 0 1]  Quaternion=[1 0 0 0]
  Spatial Contact Force6 : sm_lib/Forces and Torques/Spatial Contact Force  SenseContactBaseRotation=off  SenseContactBaseTranslation=off  CoefficientOfDynamicFriction=mu_k  CoefficientOfStaticFriction=mu_s  NormalDamping=contact_damping  NormalDampingUnits=N/(m/s)  SenseContactSignal=off  NormalStiffness=contact_stiffness  NormalStiffnessUnits=N/m  FrictionalCriticalVelocity=mu_vth  FrictionalCriticalVelocityUnits=m/s  ZeroCrossDetectContactStartAndEnd=off  SenseContactFollowerRotation=off  SenseContactFollowerTranslation=off  FrictionType=SmoothStickSlip  SenseFrictionalForceMagnitude=off  SenseNormalForceMagnitude=on  NormalForceType=SmoothSpringDamper  SenseNormalVelocity=off  SensePenetrationDepth=off  SenseSeparationDistance=off  SenseTangentialVelocity=off  NormalTransitionRegionWidth=1e-4  NormalTransitionRegionWidthUnits=m
  Sum of Elements : Sum  Inputs=+  CollapseDim=15
  G : PMIOPort  Side=Left
  B : PMIOPort  Port=2  Side=Right
  Ff : Outport
  Fn : Outport  Port=2
  wires:
  PS-Simulink Converter11/1 -> Add3/4
  PS-Simulink Converter9/1 -> Add2/4
  PS-Simulink Converter8/1 -> Add2/3
  PS-Simulink Converter5/1 -> Add2/2
  PS-Simulink Converter6/1 -> Add3/1
  Add2/1 -> Fn/1
  PS-Simulink Converter10/1 -> Add3/3
  Add3/1 -> Ff/1
  PS-Simulink Converter7/1 -> Add3/2
  Gain/1 -> Add2/1
  PS-Simulink Converter4/1 -> Sum of Elements/1
  Sum of Elements/1 -> Gain/1
  connections:
  G/RConn1 -- Spatial Contact Force6/LConn1
  Brick Solid/RConn1 -- Rigid Transform5/RConn1
  Spatial Contact Force6/RConn1 -- Point Cloud/RConn1
  B/RConn1 -- Rigid Transform2/LConn1
  Rigid Transform2/RConn1 -- Point Cloud/LConn1
  Spatial Contact Force6/RConn2 -- PS-Simulink Converter4/LConn1

== system Hector_Simulation/Hector/Left Leg/Hip Roll  ==
  joint : Inport
  Hip 2 : sm_lib/Body Elements/File Solid  ExtGeomFileName=STL files\L_hip2.STL  UnitType=Custom  ExtGeomFileUnits=m  StepReaderType=HEX  ExportConvexHullGeometry=off  InertiaType=Custom  Mass=hip2_mass  MassUnits=kg  CenterOfMass=[hip2_com_x -hip2_com_y hip2_com_z]  CenterOfMassUnits=m  MomentsOfInertia=[hip2_ixx hip2_iyy hip2_izz]  MomentsOfInertiaUnits=kg*m^2  ProductsOfInertia=[0 0 0]  ProductsOfInertiaUnits=kg*m^2  BasedOnType=Density  Density=1000  DensityUnits=kg/m^3  DoExposeReferenceFrame=on  SerializedFrames=<Frames/>  GraphicType=FromGeometry  MarkerShape=Sphere  MarkerSize=10  GraphicVisPropType=AdvancedVisualProperties  GraphicDiffuseColor=[0.9 0.9 0.9]  GraphicSpecularColor=[0.7 0.7 0.7 1.0]  GraphicAmbientColor=[0.35 0.35 0.35 1.0]  GraphicEmissiveColor=[0.0 0.0 0.0 1.0]  GraphicShininess=5  GraphicOpacity=1.0
  Hip Roll Joint : Subsystem
      settings: PortSchema="{\"entries\":[{\"content\":{\"sides\":[{\"content\":{\"connectorIds\":[\"LConn1\",\"In1\"]},\"type\":\"ConnectorPlacement.EquallySpacedRectSide\",\"uuid\":\"fe1bafd1-c1a5-4148-b465-5de294b235b8\"},{\"content\":{\"connectorIds\":[\"RConn1\",\"Out1\"],\"side\":\"RIGHT\"},\"type\":\"ConnectorPlacement.EquallySpacedRectSide\",\"uuid\":\"cbba8e06-0841-4611-b08d-047237296da9\"},{\"content\":{\"connectorIds\":[],\"side\":\"TOP\"},\"type\":\"ConnectorPlacement.EquallySpacedRectSide\",\"uuid\":\"b5035594-e8f7-4741-b410-9cfafd0751b0\"}]},\"type\":\"ConnectorPlacement.EquallySpacedConnector\",\"uuid\":\"2233606c-74e6-45bf-8a73-f401921fd730\"}],\"packageUris\":[\"http://schema.mathworks.com/mf0/Connector/R2020b\"],\"version\":\"1.0\"}"
  Rigid Transform : sm_lib/Frames and Transforms/Rigid Transform  TranslationMethod=None  TranslationStandardOffset=0  TranslationStandardOffsetUnits=m  TranslationStandardAxis=+Z  TranslationCartesianOffset=[0 0 0]  TranslationCartesianOffsetUnits=m  TranslationROffset=0  TranslationROffsetUnits=m  TranslationZOffset=0  TranslationZOffsetUnits=m  TranslationThetaOffset=0  TranslationThetaOffsetUnits=deg  RotationMethod=StandardAxis  RotationAngleUnits=deg  RotationStandardAxis=+Y  RotationAngle=90  RotationArbitraryAxis=[0 0 1]  FollAlignAxisA=+X  BaseAlignAxisA=+Y  FollAlignAxisB=+Y  BaseAlignAxisB=+Z  RotationSequenceAxes=FollowerAxes  RotationSequence=XYX  RotationSequenceAngles=[0 0 0]  RotationSequenceAnglesUnits=deg  RotationMatrix=[1 0 0; 0 1 0; 0 0 1]  Quaternion=[1 0 0 0]
  Rigid Transform1 : sm_lib/Frames and Transforms/Rigid Transform  TranslationMethod=None  TranslationStandardOffset=0  TranslationStandardOffsetUnits=m  TranslationStandardAxis=+Z  TranslationCartesianOffset=[0 0 0]  TranslationCartesianOffsetUnits=m  TranslationROffset=0  TranslationROffsetUnits=m  TranslationZOffset=0  TranslationZOffsetUnits=m  TranslationThetaOffset=0  TranslationThetaOffsetUnits=deg  RotationMethod=StandardAxis  RotationAngleUnits=deg  RotationStandardAxis=+Y  RotationAngle=-90  RotationArbitraryAxis=[0 0 1]  FollAlignAxisA=+X  BaseAlignAxisA=+Y  FollAlignAxisB=+Y  BaseAlignAxisB=+Z  RotationSequenceAxes=FollowerAxes  RotationSequence=XYX  RotationSequenceAngles=[0 0 0]  RotationSequenceAnglesUnits=deg  RotationMatrix=[1 0 0; 0 1 0; 0 0 1]  Quaternion=[1 0 0 0]
  Rigid Transform2 : sm_lib/Frames and Transforms/Rigid Transform  TranslationMethod=Cartesian  TranslationStandardOffset=0  TranslationStandardOffsetUnits=m  TranslationStandardAxis=+Z  TranslationCartesianOffset=[thigh_offset_x thigh_offset_y -thigh_offset_z]  TranslationCartesianOffsetUnits=m  TranslationROffset=0  TranslationROffsetUnits=m  TranslationZOffset=0  TranslationZOffsetUnits=m  TranslationThetaOffset=0  TranslationThetaOffsetUnits=deg  RotationMethod=None  RotationAngleUnits=deg  RotationStandardAxis=+Z  RotationAngle=90  RotationArbitraryAxis=[0 0 1]  FollAlignAxisA=+X  BaseAlignAxisA=+Y  FollAlignAxisB=+Y  BaseAlignAxisB=+Z  RotationSequenceAxes=FollowerAxes  RotationSequence=XYX  RotationSequenceAngles=[0 0 0]  RotationSequenceAnglesUnits=deg  RotationMatrix=[1 0 0; 0 1 0; 0 0 1]  Quaternion=[1 0 0 0]
  motor : sm_lib/Body Elements/File Solid  ExtGeomFileName=STL files/A1motor.STL  UnitType=Custom  ExtGeomFileUnits=m  StepReaderType=HEX  ExportConvexHullGeometry=off  InertiaType=Custom  Mass=0.605  MassUnits=kg  CenterOfMass=motor_com  CenterOfMassUnits=m  MomentsOfInertia=motor_I  MomentsOfInertiaUnits=kg*m^2  ProductsOfInertia=[0 0 0]  ProductsOfInertiaUnits=kg*m^2  BasedOnType=DensityFromFile  Density=1000  DensityUnits=kg/m^3  DoExposeReferenceFrame=on  SerializedFrames=<Frames/>  GraphicType=FromGeometry  MarkerShape=Sphere  MarkerSize=10  GraphicVisPropType=SimpleVisualProperties  GraphicDiffuseColor=[0.2 0.2 0.2]  GraphicSpecularColor=[0.5 0.5 0.5 1.0]  GraphicAmbientColor=[0.15 0.15 0.15 1.0]  GraphicEmissiveColor=[0.0 0.0 0.0 1.0]  GraphicShininess=75  GraphicOpacity=1.0
  B : PMIOPort  Side=Left
  F : PMIOPort  Port=2  Side=Right
  Sensor : Outport
  wires:
  Hip Roll Joint/1(Sensor) -> Sensor/1
  joint/1 -> Hip Roll Joint/1(joint)
  connections:
  Rigid Transform1/LConn1 -- Rigid Transform/RConn1 -- Hip Roll Joint/RConn1
  Hip Roll Joint/LConn1 -- B/RConn1
  F/RConn1 -- Rigid Transform1/RConn1
  Rigid Transform/LConn1 -- Hip 2/RConn1 -- Rigid Transform2/LConn1
  Rigid Transform2/RConn1 -- motor/RConn1

== system Hector_Simulation/Hector/Left Leg/Hip Yaw  ==
  Joint : Inport
  Hip 1 : sm_lib/Body Elements/File Solid  ExtGeomFileName=STL files\L_hip1.STL  UnitType=Custom  ExtGeomFileUnits=m  StepReaderType=HEX  ExportConvexHullGeometry=off  InertiaType=Custom  Mass=hip1_mass  MassUnits=kg  CenterOfMass=[hip1_com_x -hip1_com_y hip1_com_z]  CenterOfMassUnits=m  MomentsOfInertia=[hip1_ixx hip1_iyy hip1_izz]  MomentsOfInertiaUnits=kg*m^2  ProductsOfInertia=[0 0 0]  ProductsOfInertiaUnits=kg*m^2  BasedOnType=Density  Density=1000  DensityUnits=kg/m^3  DoExposeReferenceFrame=on  SerializedFrames=<Frames/>  GraphicType=FromGeometry  MarkerShape=Sphere  MarkerSize=10  GraphicVisPropType=AdvancedVisualProperties  GraphicDiffuseColor=[0.9 0.9 0.9]  GraphicSpecularColor=[0.7 0.7 0.7 1.0]  GraphicAmbientColor=[0.35 0.35 0.35 1.0]  GraphicEmissiveColor=[0.0 0.0 0.0 1.0]  GraphicShininess=5  GraphicOpacity=1.0
  Hip Yaw Joint : Subsystem
      settings: PortSchema="{\"entries\":[{\"content\":{\"sides\":[{\"content\":{\"connectorIds\":[\"LConn1\",\"In1\"]},\"type\":\"ConnectorPlacement.EquallySpacedRectSide\",\"uuid\":\"b3c964c5-c8eb-47b4-9e52-3baca431b477\"},{\"content\":{\"connectorIds\":[\"RConn1\",\"Out1\"],\"side\":\"RIGHT\"},\"type\":\"ConnectorPlacement.EquallySpacedRectSide\",\"uuid\":\"b5493eb8-f54f-4e30-9772-3f18358e11ff\"},{\"content\":{\"connectorIds\":[],\"side\":\"TOP\"},\"type\":\"ConnectorPlacement.EquallySpacedRectSide\",\"uuid\":\"48e308f5-e3ea-4422-818b-169dbf54879a\"}]},\"type\":\"ConnectorPlacement.EquallySpacedConnector\",\"uuid\":\"dc2c179e-5c3d-431a-a3fe-d4dab1fabc56\"}],\"packageUris\":[\"http://schema.mathworks.com/mf0/Connector/R2020b\"],\"version\":\"1.0\"}"
  Rigid Transform : sm_lib/Frames and Transforms/Rigid Transform  TranslationMethod=Cartesian  TranslationStandardOffset=0  TranslationStandardOffsetUnits=m  TranslationStandardAxis=+Z  TranslationCartesianOffset=[hip2_offset_x hip2_offset_y -hip2_offset_z]  TranslationCartesianOffsetUnits=m  TranslationROffset=0  TranslationROffsetUnits=m  TranslationZOffset=0  TranslationZOffsetUnits=m  TranslationThetaOffset=0  TranslationThetaOffsetUnits=deg  RotationMethod=StandardAxis  RotationAngleUnits=deg  RotationStandardAxis=+Z  RotationAngle=90  RotationArbitraryAxis=[0 0 1]  FollAlignAxisA=+X  BaseAlignAxisA=+Y  FollAlignAxisB=+Y  BaseAlignAxisB=+Z  RotationSequenceAxes=FollowerAxes  RotationSequence=XYX  RotationSequenceAngles=[0 0 0]  RotationSequenceAnglesUnits=deg  RotationMatrix=[1 0 0; 0 1 0; 0 0 1]  Quaternion=[1 0 0 0]
  motor : sm_lib/Body Elements/File Solid  ExtGeomFileName=STL files/A1motor.STL  UnitType=Custom  ExtGeomFileUnits=m  StepReaderType=HEX  ExportConvexHullGeometry=off  InertiaType=Custom  Mass=0.605  MassUnits=kg  CenterOfMass=motor_com  CenterOfMassUnits=m  MomentsOfInertia=motor_I  MomentsOfInertiaUnits=kg*m^2  ProductsOfInertia=[0 0 0]  ProductsOfInertiaUnits=kg*m^2  BasedOnType=DensityFromFile  Density=1000  DensityUnits=kg/m^3  DoExposeReferenceFrame=on  SerializedFrames=<Frames/>  GraphicType=FromGeometry  MarkerShape=Sphere  MarkerSize=10  GraphicVisPropType=SimpleVisualProperties  GraphicDiffuseColor=[0.2 0.2 0.2]  GraphicSpecularColor=[0.5 0.5 0.5 1.0]  GraphicAmbientColor=[0.15 0.15 0.15 1.0]  GraphicEmissiveColor=[0.0 0.0 0.0 1.0]  GraphicShininess=75  GraphicOpacity=1.0
  B : PMIOPort  Side=Left
  F : PMIOPort  Port=2  Side=Right
  Sensor : Outport
  wires:
  Joint/1 -> Hip Yaw Joint/1(Joint)
  Hip Yaw Joint/1(Sensor) -> Sensor/1
  connections:
  Hip 1/RConn1 -- F/RConn1 -- Hip Yaw Joint/RConn1 -- Rigid Transform/LConn1
  Hip Yaw Joint/LConn1 -- B/RConn1
  Rigid Transform/RConn1 -- motor/RConn1
